simulink model "Simulation_Prozessgut_11_2_2020b"  (R2020b)
settings: Solver=ode3  StartTime=0.0  StopTime=200  FixedStep=0.01  RelTol=1e-3  EnableMultiTasking=on
undefined symbols (not defined in the file): MaxFlaschen
libraries: simulink x10
settings Model: Creator=merz  LastModifiedBy=Guanran Pei
settings SolverCC: ZeroCrossAlgorithm=Non-adaptive
settings DataIOCC: LimitDataPoints=on  SaveFormat=Array  SignalLoggingSaveFormat=ModelDataLogs  ReturnWorkspaceOutputs=off  SignalLoggingName=sigsOut
settings OptimizationCC: ExpressionDepthLimit=2147483647  InitFltsAndDblsToZero=on  LifeSpan=inf
settings DebuggingCC: SaveWithParameterizedLinksMsg=none  UnderspecifiedInitializationDetection=Classic  MergeDetectMultiDrivingBlocksExec=none  SignalResolutionControl=TryResolveAllWithWarning  MultiTaskDSMMsg=warning  MultiTaskCondExecSysMsg=none  FcnCallInpInsideContextMsg=warning  StateNameClashWarn=warning  SFUnexpectedBacktrackingDiag=warning  SFNoUnconditionalDefaultTransitionDiag=warning  SFExecutionAtInitializationDiag=none  ArithmeticOperatorsInVariantConditions=warning
settings HardwareCC: ProdBitPerPointer=32  ProdBitPerSizeT=32  ProdBitPerPtrDiffT=32  ProdLargestAtomicFloat=None  ProdIntDivRoundTo=Undefined  ProdEndianess=Unspecified  ProdWordSize=32  ProdHWDeviceType=32-bit Generic  TargetUnknown=on
settings ModelReferenceCC: PropagateSignalLabelsOutOfModel=off
settings CodeAppCC: StateflowObjectComments=on
settings GRTTargetCC: TargetFcnLib=ansi_tfl_tmw.mat  TargetLangStandard=C89/C90 (ANSI)  ModelReferenceCompliant=off  CombineOutputUpdateFcns=off  MatFileLogging=off  GRTInterface=on
settings ConfigComp: CovMetricSettings=dw  CovSaveCumulativeToWorkspaceVar=on  CovSaveSingleToWorkspaceVar=on

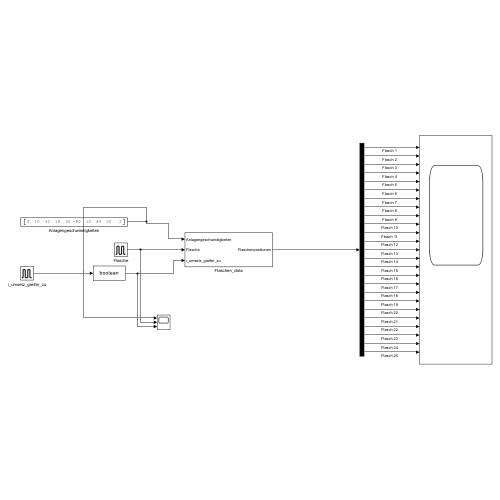
[thumbnail: Simulink's stored preview of the top-level diagram]
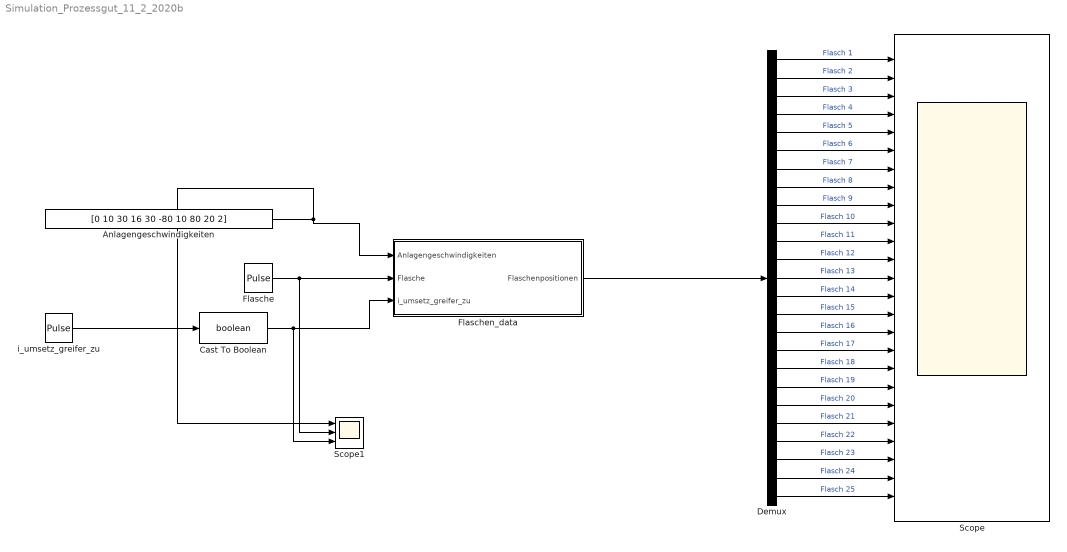
== system Simulation_Prozessgut_11_2_2020b ==
  Anlagengeschwindigkeiten : Constant  Value=[0 10 30 16 30 -80 10 80 20 2]
  Cast To Boolean : DataTypeConversion  OutDataTypeStr=boolean
  Demux : Demux  Outputs=25
  Flasche : DiscretePulseGenerator  PulseType=Time based  Period=5  PulseWidth=50
  Flaschen_data : Subsystem
  Scope : Scope  NumInputPorts=25
  Scope1 : Scope  NumInputPorts=3
  i_umsetz_greifer_zu : DiscretePulseGenerator  PulseType=Time based  Period=5  PulseWidth=50
  wires:
  Demux/19 -> Scope/19  "Flasch 19"
  Flaschen_data/1(Flaschenpositionen) -> Demux/1
  Demux/20 -> Scope/20  "Flasch 20"
  Demux/12 -> Scope/12  "Flasch 12"
  Demux/9 -> Scope/9  "Flasch 9"
  Demux/17 -> Scope/17  "Flasch 17"
  Demux/7 -> Scope/7  "Flasch 7"
  Demux/24 -> Scope/24  "Flasch 24"
  Demux/25 -> Scope/25  "Flasch 25"
  Demux/1 -> Scope/1  "Flasch 1"
  Demux/5 -> Scope/5  "Flasch 5"
  Demux/2 -> Scope/2  "Flasch 2"
  Demux/14 -> Scope/14  "Flasch 14"
  Demux/10 -> Scope/10  "Flasch 10"
  Demux/18 -> Scope/18  "Flasch 18"
  Demux/8 -> Scope/8  "Flasch 8"
  Demux/6 -> Scope/6  "Flasch 6"
  Demux/21 -> Scope/21  "Flasch 21"
  Demux/22 -> Scope/22  "Flasch 22"
  Demux/16 -> Scope/16  "Flasch 16"
  Demux/11 -> Scope/11  "Flasch 11"
  Demux/4 -> Scope/4  "Flasch 4"
  Demux/3 -> Scope/3  "Flasch 3"
  Demux/15 -> Scope/15  "Flasch 15"
  Demux/23 -> Scope/23  "Flasch 23"
  Demux/13 -> Scope/13  "Flasch 13"
  i_umsetz_greifer_zu/1 -> Cast To Boolean/1
  Anlagengeschwindigkeiten/1 -> Flaschen_data/1(Anlagengeschwindigkeiten), Scope1/1
  Flasche/1 -> Flaschen_data/2(Flasche), Scope1/2
  Cast To Boolean/1 -> Flaschen_data/3(i_umsetz_greifer_zu), Scope1/3

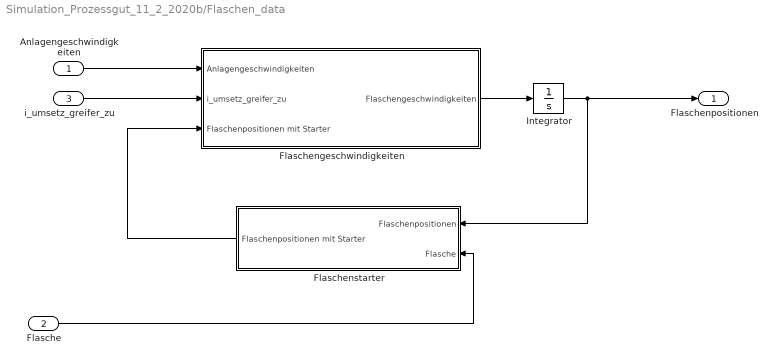
== system Simulation_Prozessgut_11_2_2020b/Flaschen_data ==
  Anlagengeschwindigkeiten : Inport
  Flasche : Inport  Port=2
  i_umsetz_greifer_zu : Inport  Port=3
  Flaschengeschwindigkeiten : Subsystem
  Flaschenstarter : Subsystem
  Integrator : Integrator
  Flaschenpositionen : Outport
  wires:
  Anlagengeschwindigkeiten/1 -> Flaschengeschwindigkeiten/1(Anlagengeschwindigkeiten)
  i_umsetz_greifer_zu/1 -> Flaschengeschwindigkeiten/2(i_umsetz_greifer_zu)
  Flasche/1 -> Flaschenstarter/2(Flasche)
  Flaschenstarter/1(Flaschenpositionen mit Starter) -> Flaschengeschwindigkeiten/3(Flaschenpositionen mit Starter)
  Flaschengeschwindigkeiten/1(Flaschengeschwindigkeiten) -> Integrator/1
  Integrator/1 -> Flaschenpositionen/1, Flaschenstarter/1(Flaschenpositionen)

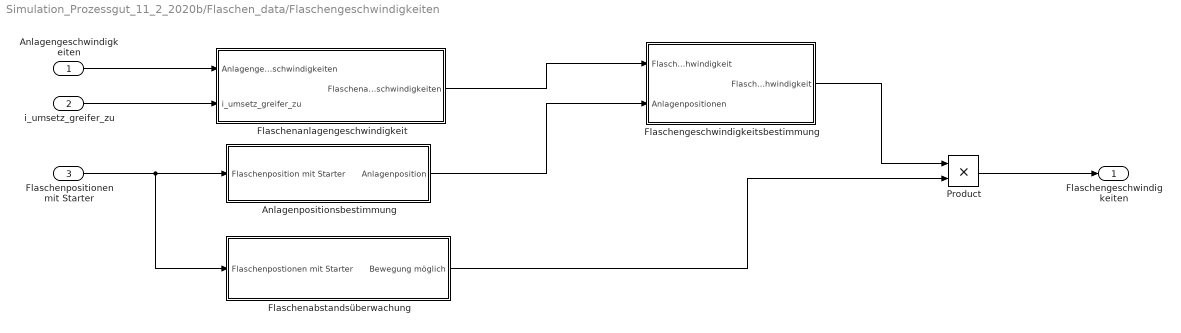
== system Simulation_Prozessgut_11_2_2020b/Flaschen_data/Flaschengeschwindigkeiten ==
  Anlagengeschwindigkeiten : Inport
  i_umsetz_greifer_zu : Inport  Port=2
  Flaschenpositionen mit Starter : Inport  Port=3
  Anlagenpositionsbestimmung : Subsystem
  Flaschenabstandsüberwachung : Subsystem
  Flaschenanlagengeschwindigkeit : Subsystem
  "Flaschengeschwindigkeitsbestimmung " : Subsystem  TreatAsAtomicUnit=on
  Product : Product
  Flaschengeschwindigkeiten : Outport
  wires:
  Anlagengeschwindigkeiten/1 -> Flaschenanlagengeschwindigkeit/1(Anlagengeschwindigkeiten)
  i_umsetz_greifer_zu/1 -> Flaschenanlagengeschwindigkeit/2(i_umsetz_greifer_zu)
  Flaschenpositionen mit Starter/1 -> Flaschenabstandsüberwachung/1(Flaschenpostionen mit Starter), Anlagenpositionsbestimmung/1(Flaschenposition mit Starter)
  Flaschenanlagengeschwindigkeit/1(Flaschenanlagengeschwindigkeiten) -> "Flaschengeschwindigkeitsbestimmung "/1(Flaschenanlagengeschwindigkeit)
  Anlagenpositionsbestimmung/1(Anlagenposition) -> "Flaschengeschwindigkeitsbestimmung "/2(Anlagenpositionen)
  "Flaschengeschwindigkeitsbestimmung "/1(Flaschengeschwindigkeit) -> Product/1
  Flaschenabstandsüberwachung/1(Bewegung möglich) -> Product/2
  Product/1 -> Flaschengeschwindigkeiten/1

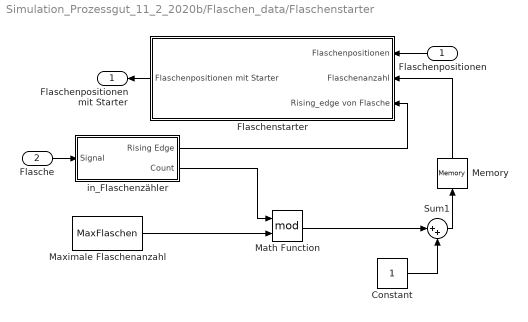
== system Simulation_Prozessgut_11_2_2020b/Flaschen_data/Flaschenstarter ==
  Flaschenpositionen : Inport
  Flasche : Inport  Port=2
  Constant : Constant  OutDataTypeStr=uint16
  Flaschenstarter : Subsystem
  Math Function : Math  Operator=mod  SignedPower=on  SaturateOnIntegerOverflow=on
  Maximale Flaschenanzahl : Constant  Value=MaxFlaschen  OutDataTypeStr=uint16
  Memory : Memory  InitialCondition=1
  Sum1 : Sum  Inputs=|++  SaturateOnIntegerOverflow=on
  in_Flaschenzähler : Subsystem
  Flaschenpositionen mit Starter : Outport
  wires:
  in_Flaschenzähler/2(Count) -> Math Function/1
  Maximale Flaschenanzahl/1 -> Math Function/2
  Math Function/1 -> Sum1/1
  in_Flaschenzähler/1(Rising Edge) -> Flaschenstarter/3(Rising_edge von Flasche)
  Sum1/1 -> Memory/1
  Constant/1 -> Sum1/2
  Memory/1 -> Flaschenstarter/2(Flaschenanzahl)
  Flaschenpositionen/1 -> Flaschenstarter/1(Flaschenpositionen)
  Flaschenstarter/1(Flaschenpositionen mit Starter) -> Flaschenpositionen mit Starter/1
  Flasche/1 -> in_Flaschenzähler/1(Signal)

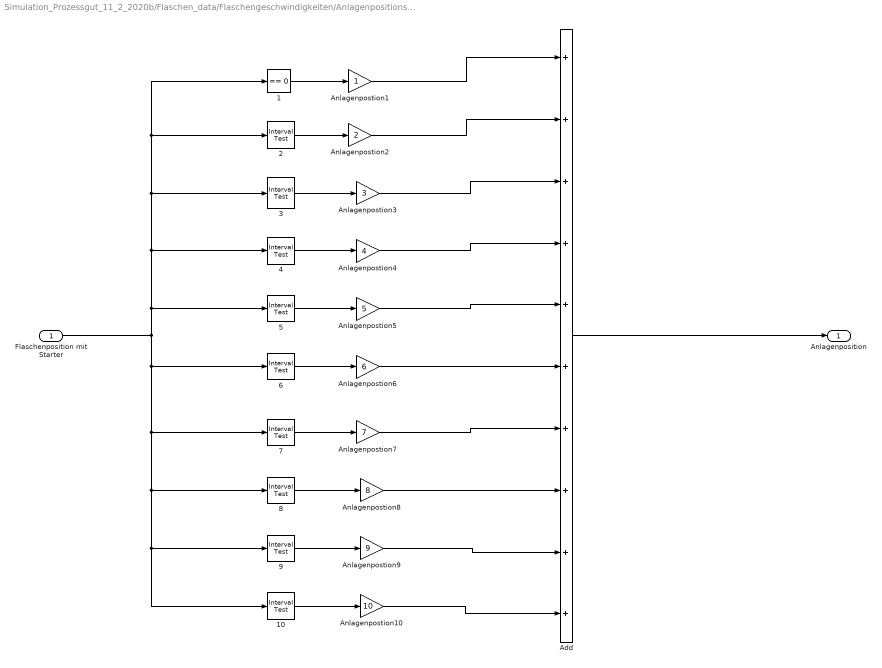
== system Simulation_Prozessgut_11_2_2020b/Flaschen_data/Flaschengeschwindigkeiten/Anlagenpositionsbestimmung ==
  Flaschenposition mit Starter : Inport
  1 : simulink/Logic and Bit Operations/Compare To Constant  relop===  const=0  OutDataTypeStr=boolean
  10 : simulink/Logic and Bit Operations/Interval Test  IntervalClosedRight=off  uplimit=inf  IntervalClosedLeft=on  lowlimit=610  OutDataTypeStr=boolean
  2 : simulink/Logic and Bit Operations/Interval Test  IntervalClosedRight=off  uplimit=101  IntervalClosedLeft=off  lowlimit=0  OutDataTypeStr=boolean
  3 : simulink/Logic and Bit Operations/Interval Test  IntervalClosedRight=off  uplimit=201  IntervalClosedLeft=on  lowlimit=101  OutDataTypeStr=boolean
  4 : simulink/Logic and Bit Operations/Interval Test  IntervalClosedRight=off  uplimit=205  IntervalClosedLeft=on  lowlimit=201  OutDataTypeStr=boolean
  5 : simulink/Logic and Bit Operations/Interval Test  IntervalClosedRight=off  uplimit=305  IntervalClosedLeft=on  lowlimit=205  OutDataTypeStr=boolean
  6 : simulink/Logic and Bit Operations/Interval Test  IntervalClosedRight=off  uplimit=405  IntervalClosedLeft=on  lowlimit=305  OutDataTypeStr=boolean
  7 : simulink/Logic and Bit Operations/Interval Test  IntervalClosedRight=off  uplimit=505  IntervalClosedLeft=on  lowlimit=405  OutDataTypeStr=boolean
  8 : simulink/Logic and Bit Operations/Interval Test  IntervalClosedRight=off  uplimit=605  IntervalClosedLeft=on  lowlimit=505  OutDataTypeStr=boolean
  9 : simulink/Logic and Bit Operations/Interval Test  IntervalClosedRight=off  uplimit=610  IntervalClosedLeft=on  lowlimit=605  OutDataTypeStr=boolean
  Add : Sum  Inputs=++++++++++
  Anlagenpostion1 : Gain
  Anlagenpostion10 : Gain  Gain=10
  Anlagenpostion2 : Gain  Gain=2
  Anlagenpostion3 : Gain  Gain=3
  Anlagenpostion4 : Gain  Gain=4
  Anlagenpostion5 : Gain  Gain=5
  Anlagenpostion6 : Gain  Gain=6
  Anlagenpostion7 : Gain  Gain=7
  Anlagenpostion8 : Gain  Gain=8
  Anlagenpostion9 : Gain  Gain=9
  Anlagenposition : Outport
  wires:
  Anlagenpostion10/1 -> Add/10
  Anlagenpostion7/1 -> Add/7
  Anlagenpostion2/1 -> Add/2
  6/1 -> Anlagenpostion6/1
  Anlagenpostion1/1 -> Add/1
  Anlagenpostion5/1 -> Add/5
  Anlagenpostion6/1 -> Add/6
  7/1 -> Anlagenpostion7/1
  9/1 -> Anlagenpostion9/1
  Anlagenpostion9/1 -> Add/9
  4/1 -> Anlagenpostion4/1
  Anlagenpostion4/1 -> Add/4
  Flaschenposition mit Starter/1 -> 3/1, 2/1, 1/1, 4/1, 5/1, 10/1, 9/1, 8/1, 7/1, 6/1
  1/1 -> Anlagenpostion1/1
  5/1 -> Anlagenpostion5/1
  Add/1 -> Anlagenposition/1
  10/1 -> Anlagenpostion10/1
  8/1 -> Anlagenpostion8/1
  2/1 -> Anlagenpostion2/1
  3/1 -> Anlagenpostion3/1
  Anlagenpostion8/1 -> Add/8
  Anlagenpostion3/1 -> Add/3

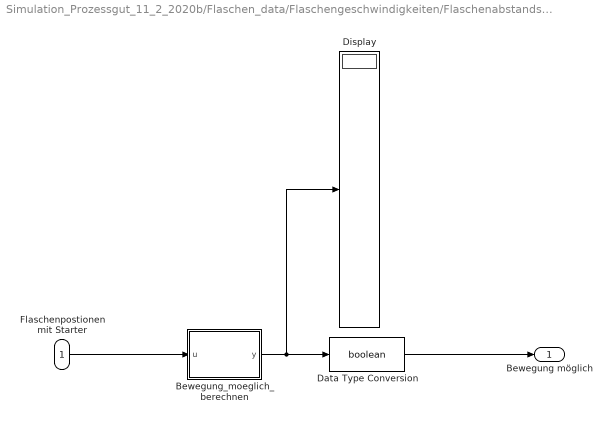
== system Simulation_Prozessgut_11_2_2020b/Flaschen_data/Flaschengeschwindigkeiten/Flaschenabstandsüberwachung ==
  Flaschenpostionen mit Starter : Inport
  Bewegung_moeglich_berechnen : MATLAB Function  TreatAsAtomicUnit=on
  Data Type Conversion : DataTypeConversion  OutDataTypeStr=boolean
  Display : Display
  Bewegung möglich : Outport
  wires:
  Bewegung_moeglich_berechnen/1(y) -> Display/1, Data Type Conversion/1
  Data Type Conversion/1 -> Bewegung möglich/1
  Flaschenpostionen mit Starter/1 -> Bewegung_moeglich_berechnen/1(u)

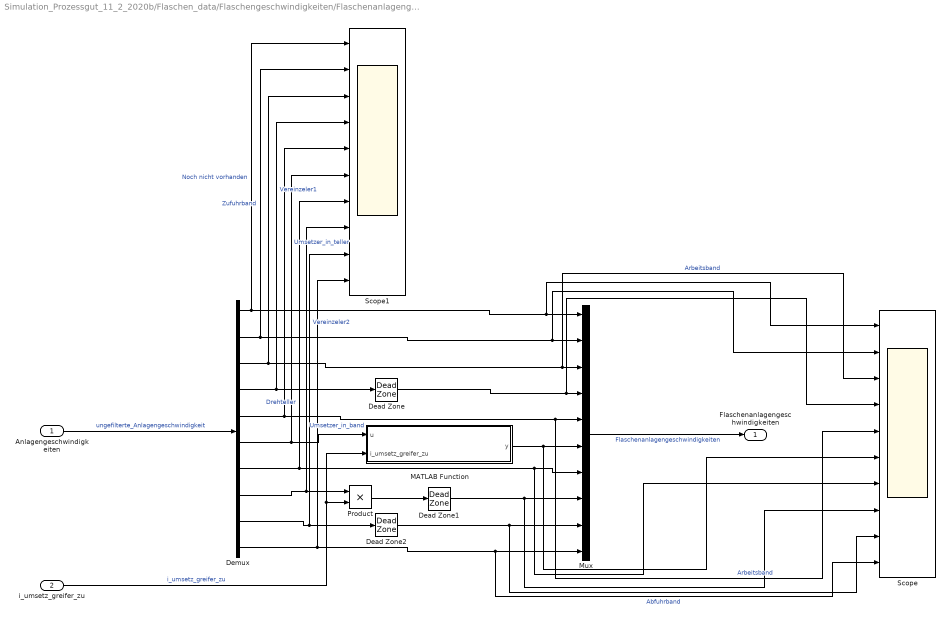
== system Simulation_Prozessgut_11_2_2020b/Flaschen_data/Flaschengeschwindigkeiten/Flaschenanlagengeschwindigkeit ==
  Anlagengeschwindigkeiten : Inport
  i_umsetz_greifer_zu : Inport  Port=2
  Dead Zone : DeadZone  LowerValue=-inf  UpperValue=0  SaturateOnIntegerOverflow=on
  Dead Zone1 : DeadZone  LowerValue=-inf  UpperValue=0  SaturateOnIntegerOverflow=on
  Dead Zone2 : DeadZone  LowerValue=-inf  UpperValue=0  SaturateOnIntegerOverflow=on
  Demux : Demux  Outputs=10
  MATLAB Function : MATLAB Function  TreatAsAtomicUnit=on
  Mux : Mux  Inputs=10
  Product : Product
  Scope : Scope  NumInputPorts=10
  Scope1 : Scope  NumInputPorts=10
  Flaschenanlagengeschwindigkeiten : Outport
  wires:
  Dead Zone2/1 -> Scope/9, Mux/9
  i_umsetz_greifer_zu/1 -> Product/2, MATLAB Function/2(i_umsetz_greifer_zu)  "i_umsetz_greifer_zu"
  Demux/3 -> Scope/3, Mux/3, Scope1/3  "Arbeitsband"
  Mux/1 -> Flaschenanlagengeschwindigkeiten/1  "Flaschenanlagengeschwindigkeiten"
  Demux/5 -> Scope1/5, Scope/5, Mux/5  "Arbeitsband"
  Dead Zone1/1 -> Scope/8, Mux/8
  Demux/10 -> Scope/10, Mux/10, Scope1/10  "Abfuhrband"
  MATLAB Function/1(y) -> Scope/6, Mux/6
  Demux/7 -> Scope1/7, Scope/7, Mux/7  "Drehteller"
  Demux/9 -> Scope1/9, Dead Zone2/1  "Vereinzeler2"
  Demux/8 -> Scope1/8, Product/1  "Umsetzer_in_band"
  Demux/2 -> Scope/2, Mux/2, Scope1/2  "Zufuhrband"
  Product/1 -> Dead Zone1/1
  Demux/4 -> Dead Zone/1, Scope1/4  "Vereinzeler1"
  Dead Zone/1 -> Scope/4, Mux/4
  Demux/6 -> Scope1/6, MATLAB Function/1(u)  "Umsetzer_in_teller"
  Demux/1 -> Scope/1, Mux/1, Scope1/1  "Noch nicht vorhanden"
  Anlagengeschwindigkeiten/1 -> Demux/1  "ungefilterte_Anlagengeschwindigkeit"

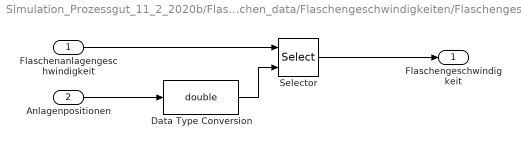
== system Simulation_Prozessgut_11_2_2020b/Flaschen_data/Flaschengeschwindigkeiten/Flaschengeschwindigkeitsbestimmung  ==
  Flaschenanlagengeschwindigkeit : Inport
  Anlagenpositionen : Inport  Port=2
  Data Type Conversion : DataTypeConversion  OutDataTypeStr=double
  Selector : Selector  InputPortWidth=10  IndexOptions=Index vector (port)  Indices=[1 3]  OutputSizes=1
  Flaschengeschwindigkeit : Outport
  wires:
  Flaschenanlagengeschwindigkeit/1 -> Selector/1
  Selector/1 -> Flaschengeschwindigkeit/1
  Anlagenpositionen/1 -> Data Type Conversion/1
  Data Type Conversion/1 -> Selector/2

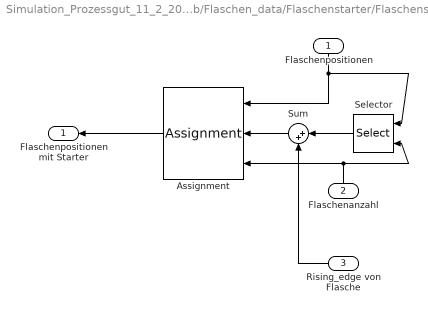
== system Simulation_Prozessgut_11_2_2020b/Flaschen_data/Flaschenstarter/Flaschenstarter ==
  Flaschenpositionen : Inport
  Flaschenanzahl : Inport  Port=2
  Rising_edge von Flasche : Inport  Port=3
  Assignment : Assignment  IndexOptions=Index vector (port)  Indices=1  OutputSizes=[1]
  Selector : Selector  InputPortWidth=MaxFlaschen  IndexOptions=Index vector (port)  Indices=[1 3]  OutputSizes=1
  Sum : Sum  Inputs=|++  OutDataTypeStr=double  RndMeth=Zero
  Flaschenpositionen mit Starter : Outport
  wires:
  Selector/1 -> Sum/1
  Sum/1 -> Assignment/2
  Flaschenanzahl/1 -> Selector/2, Assignment/3
  Flaschenpositionen/1 -> Assignment/1, Selector/1
  Assignment/1 -> Flaschenpositionen mit Starter/1
  Rising_edge von Flasche/1 -> Sum/2

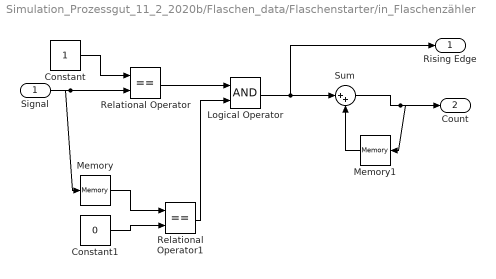
== system Simulation_Prozessgut_11_2_2020b/Flaschen_data/Flaschenstarter/in_Flaschenzähler ==
  Signal : Inport
  Constant : Constant
  Constant1 : Constant  Value=0
  Logical Operator : Logic  AllPortsSameDT=off
  Memory : Memory
  Memory1 : Memory
  Relational Operator : RelationalOperator  Operator===  RndMeth=Nearest
  Relational Operator1 : RelationalOperator  Operator===  RndMeth=Nearest
  Sum : Sum  Inputs=|++  OutDataTypeStr=uint16  SaturateOnIntegerOverflow=on
  Rising Edge : Outport
  Count : Outport  Port=2
  wires:
  Signal/1 -> Memory/1, Relational Operator/2
  Constant/1 -> Relational Operator/1
  Relational Operator/1 -> Logical Operator/1
  Constant1/1 -> Relational Operator1/2
  Memory/1 -> Relational Operator1/1
  Relational Operator1/1 -> Logical Operator/2
  Logical Operator/1 -> Sum/1, Rising Edge/1
  Memory1/1 -> Sum/2
  Sum/1 -> Count/1, Memory1/1

== matlab function Simulation_Prozessgut_11_2_2020b/Flaschen_data/Flaschengeschwindigkeiten/Flaschenanlagengeschwindigkeit/MATLAB Function ==
  data: u input; y output; i_umsetz_greifer_zu input
function y = fcn(u,i_umsetz_greifer_zu)

y = 0.5*(abs(u)-u)*i_umsetz_greifer_zu;

== matlab function Simulation_Prozessgut_11_2_2020b/Flaschen_data/Flaschengeschwindigkeiten/Flaschenabstandsüberwachung/Bewegung_moeglich_berechnen ==
  data: u input; y output
function y = fcn(u)
Flaschenabstand = circshift(u,1) - u;
y = zeros(1,25);
for i = 1:length(Flaschenabstand)
    if(Flaschenabstand(i)<6)
        y(i) = 0;
    else
        y(i) = 1;
    end
end
y(1) = 1;
